simulink model "Experiment_4_1_Plant"  (R2018a)
settings: Solver=ode8  StartTime=0.0  StopTime=inf  FixedStep=Ts  RelTol=1e-8  AbsTol=1e-8  EnableMultiTasking=on
values from neighbouring files (symbols this model uses):
  L = y    [plotfft.m]
undefined symbols (not defined in the file or in its folder): epsilon, K, m, R, theta_0, theta_dot_0
libraries: EEE481Arduino x2
settings Model: ExtModeTrigDuration=2  Creator=vaggarw7  LastModifiedBy=abhig
settings SolverCC: AutoScaleAbsTol=off
settings OptimizationCC: PassReuseOutputArgsAs=Individual arguments  MaxStackSize=64
settings DebuggingCC: ParameterTunabilityLossMsg=error
settings HardwareCC: ProdBitPerPointer=32  ProdBitPerSizeT=32  ProdBitPerPtrDiffT=32  ProdLargestAtomicInteger=Long  ProdLargestAtomicFloat=Double  ProdWordSize=32  ProdHWDeviceType=ARM Compatible->ARM Cortex
settings SFSimCC: MATLABDynamicMemAlloc=off
settings RTWCC: SystemTargetFile=ert.tlc  HardwareBoard=Arduino Due  TLCOptions=-aInlineSetEventsForThisBaseRateFcn=TLC_FALSE -aSuppressMultiTaskScheduler=TLC_FALSE -aRateBasedStepFcn=1  TemplateMakefile=ert_default_tmf  GenerateReport=on  Toolchain=Arduino ARM  BuildConfiguration=Faster Runs  IncludeHyperlinkInReport=on  LaunchReport=on  GenerateTraceInfo=on  GenerateTraceReport=on  GenerateTraceReportSl=on  GenerateTraceReportSf=on  GenerateTraceReportEml=on
settings CodeAppCC: ForceParamTrailComments=on  IgnoreCustomStorageClasses=off  OperatorAnnotations=on  SimulinkDataObjDesc=on  SFDataObjDesc=on  MATLABFcnDesc=on  InsertBlockDesc=on  StateflowObjectComments=on  MATLABSourceComments=on
settings ERTTargetCC: SupportContinuousTime=on  SupportVariableSizeSignals=on

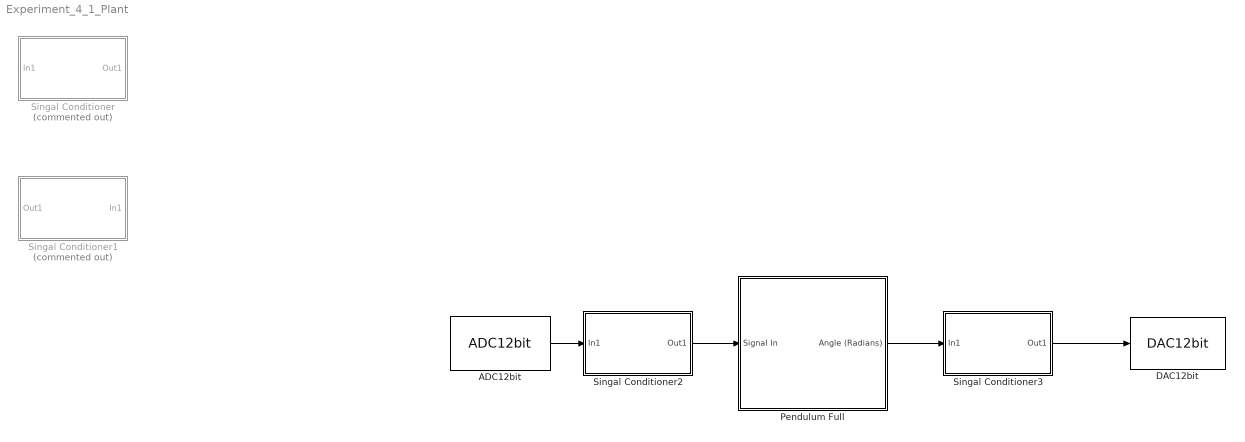
== system Experiment_4_1_Plant ==
  ADC12bit : EEE481Arduino/ADC12bit  pinNum=0  Tsa=Ts
      settings: SourceProductName=EEE 481 Arduino
  DAC12bit : EEE481Arduino/DAC12bit  Tsa=Ts  DACNum=0
      settings: SourceProductName=EEE 481 Arduino
  Pendulum Full : Subsystem
  Singal Conditioner : Subsystem  Commented=on  mask{out_min=0.56, out_max=2.76, in_min=-1, in_max=3}
      mask prompts: out_min "Minimum Value of Output Signal"; out_max "Maximum Value of Output Signal"; in_min "Minimum Value of Input Signal"; in_max "Maximum Value of Input Signal"
  Singal Conditioner1 : Subsystem  Commented=on  mask{out_min=0.56, out_max=2.76, in_min=-1, in_max=3}
      mask prompts: out_min "Minimum Value of Output Signal"; out_max "Maximum Value of Output Signal"; in_min "Minimum Value of Input Signal"; in_max "Maximum Value of Input Signal"
  Singal Conditioner2 : Subsystem  mask{out_min=-255, out_max=255, in_min=0.56, in_max=2.76}
      mask prompts: out_min "Minimum Value of Output Signal"; out_max "Maximum Value of Output Signal"; in_min "Minimum Value of Input Signal"; in_max "Maximum Value of Input Signal"
  Singal Conditioner3 : Subsystem  mask{out_min=0.56, out_max=2.76, in_min=-pi/2, in_max=pi/2}
      mask prompts: out_min "Minimum Value of Output Signal"; out_max "Maximum Value of Output Signal"; in_min "Minimum Value of Input Signal"; in_max "Maximum Value of Input Signal"
  wires:
  Pendulum Full/1(Angle (Radians)) -> Singal Conditioner3/1(In1)
  ADC12bit/1 -> Singal Conditioner2/1(In1)
  Singal Conditioner2/1(Out1) -> Pendulum Full/1(Signal In)
  Singal Conditioner3/1(Out1) -> DAC12bit/1

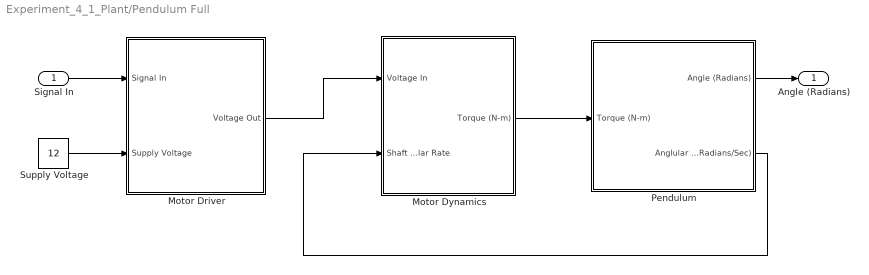
== system Experiment_4_1_Plant/Pendulum Full ==
  Signal In : Inport
  Motor Driver : Subsystem
  Motor Dynamics : Subsystem  mask{K=K, R=R}
      mask prompts: K "Motor Constant"; R "Motor Armature Resistance (Ohms)"
  Pendulum : Subsystem  mask{m=m, L=L, epsilon=epsilon, g=9.81, theta=theta_0, theta_dot=theta_dot_0}
      mask prompts: m "Mass of Bob (Kg)"; L "Length of arm (m)"; epsilon "Friction Coefficient"; g "Acceleration due to Gravity (m/s/s)"; theta "Angle Initial Condition (Radians)"; theta_dot "Anglular Rate Initial Condition (Radians/Sec)"
  Supply Voltage : Constant  Value=12
  Angle (Radians) : Outport  OutputWhenDisabled=reset  InitialOutput=0
  wires:
  Supply Voltage/1 -> Motor Driver/2(Supply Voltage)
  Pendulum/1(Angle (Radians)) -> Angle (Radians)/1
  Motor Dynamics/1(Torque (N-m)) -> Pendulum/1("Torque (N-m) ")
  Pendulum/2(Anglular Rate (Radians/Sec)) -> Motor Dynamics/2(Shaft Angular Rate)
  Signal In/1 -> Motor Driver/1(Signal In)
  Motor Driver/1(Voltage Out) -> Motor Dynamics/1(Voltage In)

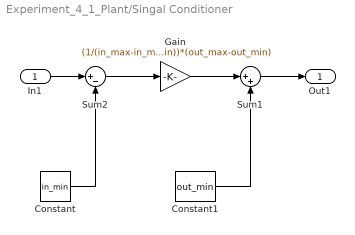
== system Experiment_4_1_Plant/Singal Conditioner ==
  In1 : Inport
  Constant : Constant  Value=in_min
  Constant1 : Constant  Value=out_min
  Gain : Gain  Gain=(1/(in_max-in_min))*(out_max-out_min)
  Sum1 : Sum  Inputs=|++
  Sum2 : Sum  Inputs=|+-
  Out1 : Outport
  wires:
  Sum2/1 -> Gain/1
  In1/1 -> Sum2/1
  Constant1/1 -> Sum1/2
  Sum1/1 -> Out1/1
  Gain/1 -> Sum1/1
  Constant/1 -> Sum2/2

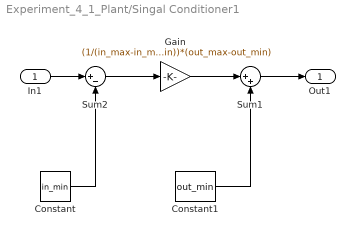
== system Experiment_4_1_Plant/Singal Conditioner1 ==
  In1 : Inport
  Constant : Constant  Value=in_min
  Constant1 : Constant  Value=out_min
  Gain : Gain  Gain=(1/(in_max-in_min))*(out_max-out_min)
  Sum1 : Sum  Inputs=|++
  Sum2 : Sum  Inputs=|+-
  Out1 : Outport
  wires:
  Constant/1 -> Sum2/2
  Gain/1 -> Sum1/1
  Sum1/1 -> Out1/1
  Constant1/1 -> Sum1/2
  In1/1 -> Sum2/1
  Sum2/1 -> Gain/1

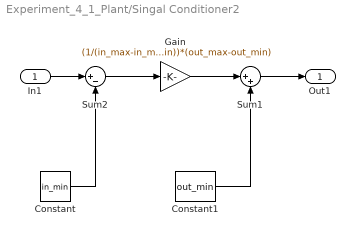
== system Experiment_4_1_Plant/Singal Conditioner2 ==
  In1 : Inport
  Constant : Constant  Value=in_min
  Constant1 : Constant  Value=out_min
  Gain : Gain  Gain=(1/(in_max-in_min))*(out_max-out_min)
  Sum1 : Sum  Inputs=|++
  Sum2 : Sum  Inputs=|+-
  Out1 : Outport
  wires:
  Sum2/1 -> Gain/1
  In1/1 -> Sum2/1
  Constant1/1 -> Sum1/2
  Sum1/1 -> Out1/1
  Gain/1 -> Sum1/1
  Constant/1 -> Sum2/2

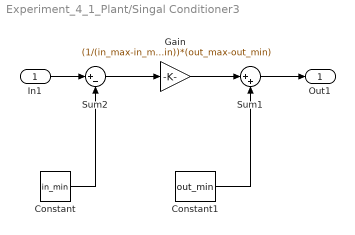
== system Experiment_4_1_Plant/Singal Conditioner3 ==
  In1 : Inport
  Constant : Constant  Value=in_min
  Constant1 : Constant  Value=out_min
  Gain : Gain  Gain=(1/(in_max-in_min))*(out_max-out_min)
  Sum1 : Sum  Inputs=|++
  Sum2 : Sum  Inputs=|+-
  Out1 : Outport
  wires:
  Constant/1 -> Sum2/2
  Gain/1 -> Sum1/1
  Sum1/1 -> Out1/1
  Constant1/1 -> Sum1/2
  In1/1 -> Sum2/1
  Sum2/1 -> Gain/1

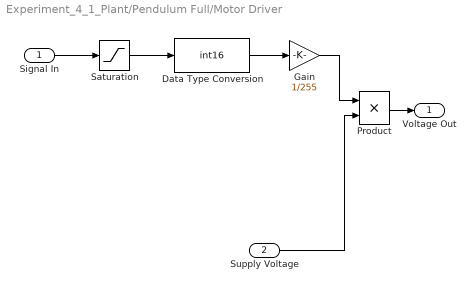
== system Experiment_4_1_Plant/Pendulum Full/Motor Driver ==
  Signal In : Inport
  Supply Voltage : Inport  Port=2
  Data Type Conversion : DataTypeConversion  OutDataTypeStr=int16
  Gain : Gain  Gain=1/255
  Product : Product
  Saturation : Saturate  UpperLimit=255  LowerLimit=-255
  Voltage Out : Outport
  wires:
  Gain/1 -> Product/1
  Data Type Conversion/1 -> Gain/1
  Saturation/1 -> Data Type Conversion/1
  Supply Voltage/1 -> Product/2
  Product/1 -> Voltage Out/1
  Signal In/1 -> Saturation/1

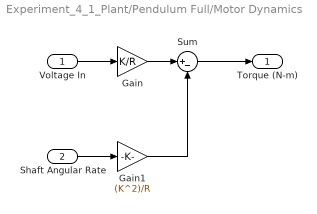
== system Experiment_4_1_Plant/Pendulum Full/Motor Dynamics ==
  Voltage In : Inport
  Shaft Angular Rate : Inport  Port=2
  Gain : Gain  Gain=K/R
  Gain1 : Gain  Gain=(K^2)/R
  Sum : Sum  Inputs=|+-
  Torque (N-m) : Outport
  wires:
  Shaft Angular Rate/1 -> Gain1/1
  Sum/1 -> Torque (N-m)/1
  Gain1/1 -> Sum/2
  Voltage In/1 -> Gain/1
  Gain/1 -> Sum/1

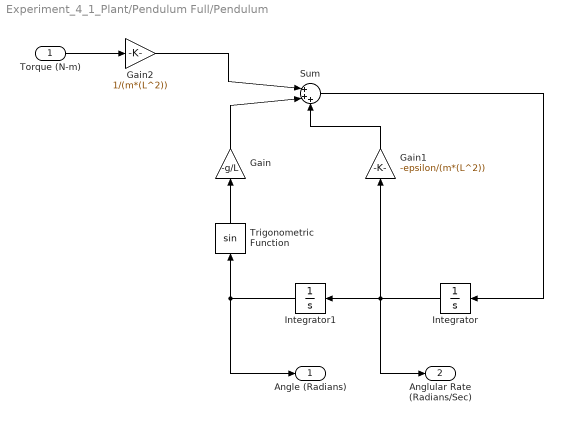
== system Experiment_4_1_Plant/Pendulum Full/Pendulum ==
  "Torque (N-m) " : Inport
  Gain : Gain  Gain=-g/L
  Gain1 : Gain  Gain=-epsilon/(m*(L^2))
  Gain2 : Gain  Gain=1/(m*(L^2))
  Integrator : Integrator  InitialCondition=theta_dot
  Integrator1 : Integrator  InitialCondition=theta
  Sum : Sum  Inputs=|+++
  Trigonometric Function : Trigonometry
  Angle (Radians) : Outport
  Anglular Rate (Radians/Sec) : Outport  Port=2
  wires:
  Integrator1/1 -> Angle (Radians)/1, Trigonometric Function/1
  Integrator/1 -> Anglular Rate (Radians/Sec)/1, Gain1/1, Integrator1/1
  Gain1/1 -> Sum/3
  Trigonometric Function/1 -> Gain/1
  "Torque (N-m) "/1 -> Gain2/1
  Sum/1 -> Integrator/1
  Gain2/1 -> Sum/1
  Gain/1 -> Sum/2
